simulink model "SinglePendDisturbance"  (R2025b)
settings: Solver=FixedStepAuto  StartTime=0  StopTime=10  FixedStep=0.02  MaxStep=0.02  RelTol=1e-3  AbsTol=1e-6
undefined symbols (not defined in the file): b, g, K, L, m, M
libraries: simulink x1
CloseFcn:
  | set(groot,'ShowHiddenHandles','on');
  | c = get(groot,'Children');
  | close(c);
  | clear c;
  | set(groot,'ShowHiddenHandles','off');
Description:
  | Inverted Pendulum with Animation
  | 
  | This example shows how to model an inverted pendulum.  The animation is created using MATLAB(R) Handle Graphics(R).  The animation block is a masked
  | S-function.  For more information, use the context menu to look under the Animation block's mask
  | and open the S-function for editing.
settings Model: PacingRate=0.320000  ExtModeAutoUpdateStatusClock=off  Creator=The MathWorks, Inc.  LastModifiedBy=lucas
settings SolverCC: AutoScaleAbsTol=off  AlgebraicLoopSolver=TrustRegion
settings DataIOCC: ExternalInput=[]  InitialState=[]  SaveFormat=Array  SaveOutput=off  SaveTime=off
settings OptimizationCC: BlockReduction=off  BooleanDataType=off  ReuseModelBlockBuffer=off  ExpressionDepthLimit=2147483647.0  InitFltsAndDblsToZero=on  LifeSpan=inf
settings DebuggingCC: SaveWithParameterizedLinksMsg=none  UnderspecifiedInitializationDetection=Classic  MergeDetectMultiDrivingBlocksExec=none  SignalResolutionControl=TryResolveAllWithWarning  MultiTaskDSMMsg=warning  MultiTaskCondExecSysMsg=none  SigSpecEnsureSampleTimeMsg=none  FcnCallInpInsideContextMsg=warning  UnconnectedInputMsg=warning  UnconnectedOutputMsg=warning  UnconnectedLineMsg=warning  StateNameClashWarn=warning  SubsystemReferenceDiagnosticForUnitTest=warning  SFUnexpectedBacktrackingDiag=warning  SFNoUnconditionalDefaultTransitionDiag=warning  SFExecutionAtInitializationDiag=none  ArithmeticOperatorsInVariantConditions=warning
settings HardwareCC: ProdBitPerPointer=32.0  ProdBitPerSizeT=32.0  ProdBitPerPtrDiffT=32.0  ProdLargestAtomicFloat=None  ProdIntDivRoundTo=Undefined  ProdEndianess=Unspecified  ProdWordSize=32.0  ProdHWDeviceType=32-bit Generic  TargetUnknown=on
settings ModelReferenceCC: EnableRefExpFcnMdlSchedulingChecks=on  PropagateSignalLabelsOutOfModel=off
settings SFSimCC: SimUseLocalCustomCode=off  CustomCodeUndefinedFunction=UseInterfaceOnly
settings RTWCC: RTWUseLocalCustomCode=off  GPUComputeCapability=3.5
settings CodeAppCC: StateflowObjectComments=on
settings GRTTargetCC: TargetFcnLib=ansi_tfl_tmw.mat  TargetLangStandard=C89/C90 (ANSI)  CombineOutputUpdateFcns=off  GRTInterface=on
settings ConfigComp: CovMetricSettings=dw  CovSaveCumulativeToWorkspaceVar=on  CovSaveSingleToWorkspaceVar=on  CovExternalEMLEnable=off
settings SimscapeCC: SimscapeLogDataHistory=5000  SimscapeLogDecimation=1

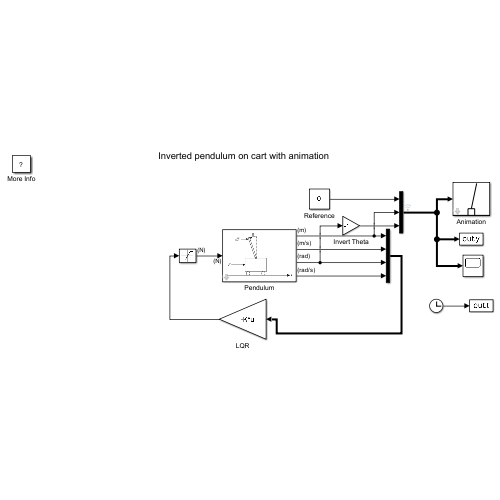
[thumbnail: Simulink's stored preview of the top-level diagram]
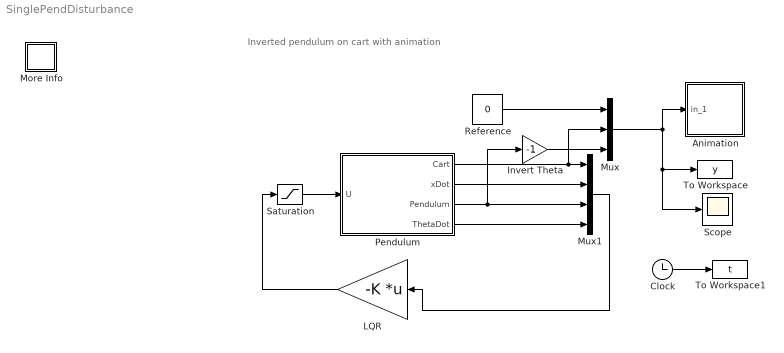
== system SinglePendDisturbance ==
  note: Inverted pendulum on cart with animation
  Animation : Subsystem  mask(Pendulum plot){RefBlock=Reference}
      mask prompts: RefBlock "DC reference signal block name:"
      mask help: Pendulum plot
      mask Help: Pendulum animation function using Handle graphics.
      mask Display: plot([-10 10],[0 0],[-2 -2 2 2],[0 1 1 0],[0 3],[1 5])
  Clock : Clock
  Invert Theta : Gain  Gain=-1
  LQR : Gain  Gain=-K  Multiplication=Matrix(K*u)
  More Info : Subsystem
      settings: OpenFcn=showExample('simulink_general/penddemoExample')
      mask Display: disp('?')
  Mux : Mux  Inputs=3
  Mux1 : Mux
  Pendulum : Subsystem  mask(Inverted Pendulum Dynamics){Mcart=M, m=m, l=L, g=g, b=b}
      mask prompts: Mcart "Mass of cart (kg):"; m "Mass of pendulum (kg):"; l "Distance to pendulum center of mass (m):"; g "Acceleration of gravity (m/s^2):"; b "Friction coef"
      mask help: Masked subsystem containing nonlinear dynamics of inverted pendulum on a cart.
      mask Help: Nonlinear dynamics of inverted pendulum on cart.
      mask Display: image('pendulum1.png');
  Reference : Constant  Value=0
  Saturation : Saturate  UpperLimit=10  LowerLimit=-10
  Scope : Scope
      settings: ActiveDisplayYMinimum=-2.23423011012781  ActiveDisplayYMaximum=1.5815811233475343  YLabel=Refernce and Cart Position (m), Pendulum Position (rad)
  To Workspace : ToWorkspace  VariableName=y  SampleTime=0.1
  To Workspace1 : ToWorkspace  VariableName=t  SampleTime=0.1
  wires:
  Mux/1 -> Scope/1, To Workspace/1, Animation/1(in_1)
  LQR/1 -> Saturation/1
  Saturation/1 -> Pendulum/1(U)
  Clock/1 -> To Workspace1/1
  Pendulum/1(Cart) -> Mux1/1, Mux/2
  Reference/1 -> Mux/1
  Mux1/1 -> LQR/1
  Pendulum/2(xDot) -> Mux1/2
  Invert Theta/1 -> Mux/3
  Pendulum/4(ThetaDot) -> Mux1/4
  Pendulum/3(Pendulum) -> Invert Theta/1, Mux1/3

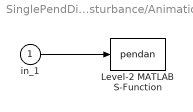
== system SinglePendDisturbance/Animation ==
  in_1 : Inport
  Level-2 MATLAB S-Function : M-S-Function  FunctionName=pendan  Parameters=RefBlock
  wires:
  in_1/1 -> Level-2 MATLAB S-Function/1

== system SinglePendDisturbance/More Info ==

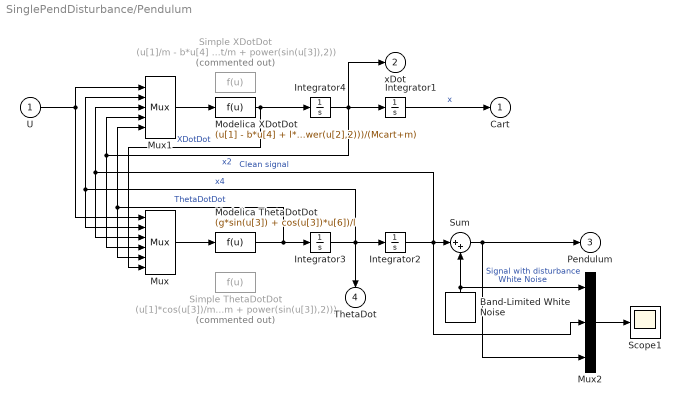
== system SinglePendDisturbance/Pendulum ==
  U : Inport  Unit=N
  Band-Limited White Noise : simulink/Sources/Band-Limited White Noise  Cov=[0.0001]  Ts=0.02  seed=[23341]
  Integrator1 : Integrator  InitialCondition=1.2  ContinuousStateAttributes='CartPosition'
  Integrator2 : Integrator  InitialCondition=.27  ContinuousStateAttributes='PendulumAngle'
  Integrator3 : Integrator  InitialCondition=.5  ContinuousStateAttributes='PendulumAngularVelocity'
  Integrator4 : Integrator  ContinuousStateAttributes='CartVelocity'
  Modelica ThetaDotDot : Fcn  Expr=(g*sin(u[3]) + cos(u[3])*u[6])/l
  Modelica XDotDot : Fcn  Expr=(u[1] - b*u[4] + l*m*(cos(u[3])*u[5] - sin(u[3])*power(u[2],2)))/(Mcart+m)
  Mux : Mux  Inputs=6
  Mux1 : Mux  Inputs=5
  Mux2 : Mux  Inputs=3
  Scope1 : Scope
      settings: ActiveDisplayYMinimum=-0.14664935477454569  ActiveDisplayYMaximum=0.20865363080540175
  Simple ThetaDotDot : Fcn  Commented=on  Expr=(u[1]*cos(u[3])/m + Mcart*g*sin(u[3])/m - l*power(u[2],2)*sin(u[3])*cos(u[3]))/(l*(Mcart/m + power(sin(u[3]),2)))
  Simple XDotDot : Fcn  Commented=on  Expr=(u[1]/m - b*u[4] + g*sin(u[3])*cos(u[3]) - l*power(u[2],2)*sin(u[3]))/(Mcart/m + power(sin(u[3]),2))
  Sum : Sum  Inputs=|++
  Cart : Outport  Unit=m  InitialOutput=0  VectorParamsAs1DForOutWhenUnconnected=off
  xDot : Outport  Port=2  Unit=m/s  InitialOutput=0  VectorParamsAs1DForOutWhenUnconnected=off
  Pendulum : Outport  Port=3  Unit=rad  InitialOutput=0  VectorParamsAs1DForOutWhenUnconnected=off
  ThetaDot : Outport  Port=4  Unit=rad/s  InitialOutput=0  VectorParamsAs1DForOutWhenUnconnected=off
  wires:
  Integrator4/1 -> Mux1/4, Mux/4, Integrator1/1, xDot/1  "x2"
  U/1 -> Mux1/1, Mux/1
  Integrator3/1 -> Mux1/2, Mux/2, Integrator2/1, ThetaDot/1  "x4"
  Modelica XDotDot/1 -> Mux/6, Integrator4/1  "XDotDot"
  Modelica ThetaDotDot/1 -> Mux1/5, Mux/5, Integrator3/1  "ThetaDotDot"
  Band-Limited White Noise/1 -> Sum/2, Mux2/1  "White Noise"
  Mux2/1 -> Scope1/1
  Sum/1 -> Mux2/3, Pendulum/1  "Signal with disturbance"
  Integrator2/1 -> Sum/1, Mux2/2, Mux1/3, Mux/3  "Clean signal"
  Mux1/1 -> Modelica XDotDot/1
  Mux/1 -> Modelica ThetaDotDot/1
  Integrator1/1 -> Cart/1  "x"
